simulink model "forloopeml"  (Simulink 7.1)
settings: Solver=FixedStepDiscrete  StartTime=0.0  StopTime=10.0  FixedStep=.01  RelTol=1e-3
settings Model: Creator=ajayaram  LastModifiedBy=ajayaram
settings OptimizationCC: InlineParams=on  OptimizeModelRefInitCode=on  LifeSpan=1
settings DebuggingCC: SaveWithParameterizedLinksMsg=none
settings RTWCC: SystemTargetFile=ert.tlc  GenCodeOnly=on  GenerateMakefile=off  TemplateMakefile=ert_default_tmf  Description=Real-Time Workshop Embedded Coder (no auto configuration)  GenerateReport=on  ProcessScript=ert_make_rtw_hook  IncludeHyperlinkInReport=on  LaunchReport=on
settings CodeAppCC: GenerateComments=off  IgnoreCustomStorageClasses=off  SimulinkBlockComments=off
settings ERTTargetCC: TargetFcnLib=ansi_tfl_tmw.mat  InlinedParameterPlacement=NonHierarchical  ERTCustomFileTemplate=example_file_process.tlc

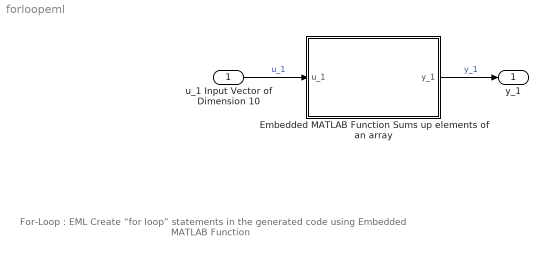
== system forloopeml ==
  note: For-Loop : EML
      | Create “for loop” statements in the generated
      | code using Embedded MATLAB Function
  u_1 Input Vector of Dimension 10 : Inport  PortDimensions=10  OutDataType=sfix(16)  OutScaling=2^0
  Embedded MATLAB Function Sums up elements of an array : Stateflow chart
  y_1 : Outport  OutDataType=sfix(16)  OutScaling=2^0
  wires:
  Embedded MATLAB Function Sums up elements of an array/1(y_1) -> y_1/1  "y_1"
  u_1 Input Vector of Dimension 10/1 -> Embedded MATLAB Function Sums up elements of an array/1(u_1)  "u_1"

== matlab function Embedded MATLAB Function Sums up elements of an array ==
  data: u_1 input double; y_1 output double
function y_1 = fcn(u_1)

% NOTE: In M-Script, the index variable varies from 1 through 10


y_1 = 0;

for inx=1:10
    y_1 = u_1(inx) + y_1 ;
end
